simulink model "DecoupledControl"  (R2022a)
settings: Solver=VariableStepAuto  StartTime=0.0  StopTime=30  MaxStep=0.0001  RelTol=1e-3
undefined symbols (not defined in the file): K1, K2, N1, N2, q01, q02, tau0
settings Model: Creator=y.briere  LastModifiedBy=fades
settings DebuggingCC: UnconnectedInputMsg=warning  UnconnectedOutputMsg=warning  UnconnectedLineMsg=warning
settings RTWCC: DLArmComputeVersion=19.05

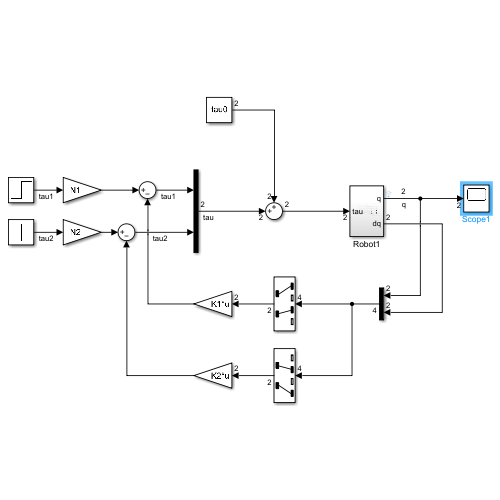
[thumbnail: Simulink's stored preview of the top-level diagram]
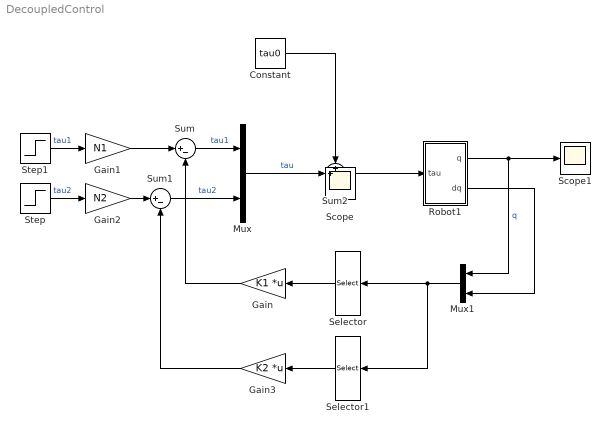
== system DecoupledControl ==
  Constant : Constant  Value=tau0
  Gain : Gain  Gain=K1  Multiplication=Matrix(K*u)
  Gain1 : Gain  Gain=N1
  Gain2 : Gain  Gain=N2
  Gain3 : Gain  Gain=K2  Multiplication=Matrix(K*u)
  Mux : Mux  Inputs=2
  Mux1 : Mux  Inputs=2
  Robot1 : Subsystem
  Scope1 : Scope
  Selector : Selector  InputPortWidth=4  IndexOptions=Index vector (dialog)  Indices=[1 3]  OutputSizes=1
  Selector1 : Selector  InputPortWidth=4  IndexOptions=Index vector (dialog)  Indices=[2 4]  OutputSizes=1
  Step : Step  Time=10  Before=q02  After=q02 + pi/2  SampleTime=0
  Step1 : Step  Before=q01  After=q01  SampleTime=0
  Sum : Sum  Inputs=|+-
  Sum1 : Sum  Inputs=|+-
  Sum2 : Sum  Inputs=++|
  Scope : Scope
  wires:
  Sum1/1 -> Mux/2  "tau2"
  Sum/1 -> Mux/1  "tau1"
  Robot1/1(q) -> Mux1/1, Scope1/1  "q"
  Selector/1 -> Gain/1
  Step1/1 -> Gain1/1  "tau1"
  Step/1 -> Gain2/1  "tau2"
  Gain2/1 -> Sum1/1
  Selector1/1 -> Gain3/1
  Gain/1 -> Sum/2
  Gain3/1 -> Sum1/2
  Mux1/1 -> Selector1/1, Selector/1
  Robot1/2(dq) -> Mux1/2
  Gain1/1 -> Sum/1
  Constant/1 -> Sum2/1
  Sum2/1 -> Robot1/1(tau)
  Mux/1 -> Sum2/2  "tau"

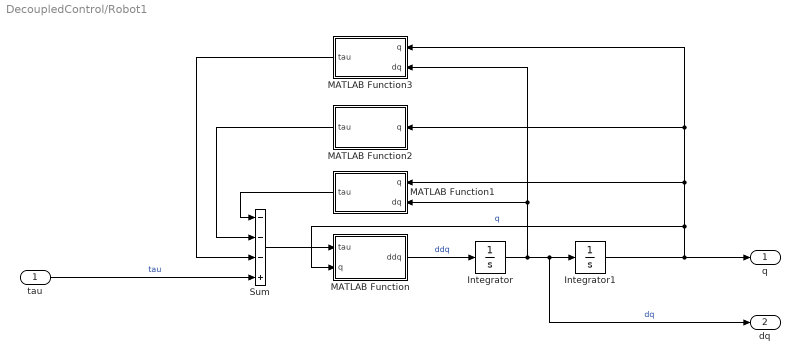
== system DecoupledControl/Robot1 ==
  tau : Inport
  Integrator : Integrator  InitialCondition=[0:0]
  Integrator1 : Integrator  InitialCondition=[q01;q02]
  MATLAB Function : MATLAB Function  TreatAsAtomicUnit=on
  MATLAB Function1 : MATLAB Function  TreatAsAtomicUnit=on
  MATLAB Function2 : MATLAB Function  TreatAsAtomicUnit=on
  MATLAB Function3 : MATLAB Function  TreatAsAtomicUnit=on
  Sum : Sum  Inputs=---+
  q : Outport
  dq : Outport  Port=2
  wires:
  Integrator/1 -> MATLAB Function3/2(dq), MATLAB Function1/2(dq), dq/1, Integrator1/1  "dq"
  Integrator1/1 -> MATLAB Function3/1(q), MATLAB Function2/1(q), MATLAB Function1/1(q), MATLAB Function/2(q), q/1  "q"
  MATLAB Function3/1(tau) -> Sum/3
  MATLAB Function/1(ddq) -> Integrator/1  "ddq"
  Sum/1 -> MATLAB Function/1(tau)
  MATLAB Function1/1(tau) -> Sum/1
  MATLAB Function2/1(tau) -> Sum/2
  tau/1 -> Sum/4  "tau"

== matlab function DecoupledControl/Robot1/MATLAB Function ==
  data: tau input; q input; ddq output
function ddq  = invM(tau,q)
% Mass matrix
R.m1 = 1; % Arm 1 mass
R.m2 = 1; % Arm 2 mass
R.L1 = 1; % Arm 1 length
R.L2 = 1; % Arm 2 length
M = [(R.m1*R.L1^2)/4+R.m2*(R.L1^2+R.L2^2/4+R.L1*R.L2*cos(q(2))) ,  R.m2*R.L2*(R.L2+ 2*R.L1*cos(q(2)))/4
    R.m2*R.L2*(R.L2+ 2*R.L1*cos(q(2)))/4                       ,  R.m2*R.L2^2/4];

ddq = M\tau;

== matlab function DecoupledControl/Robot1/MATLAB Function1 ==
  data: q input; dq input; tau output
function tau  = coriolis(q,dq)
% Convective Matrix
%Robot parameters
R.m1 = 1; % Arm 1 mass
R.m2 = 1; % Arm 2 mass
R.L1 = 1; % Arm 1 length
R.L2 = 1; % Arm 2 length
Cm = [-R.m2*R.L1*R.L2*sin(q(2))*dq(2) -R.m2*R.L1*R.L2*sin(q(2))/2*dq(2);...
    R.m2*R.L1*R.L2*dq(1)*sin(q(2))/2 0];
tau = Cm*dq;

== matlab function DecoupledControl/Robot1/MATLAB Function2 ==
  data: q input; tau output
function tau  = gravity(q)
%Robot parameters
R.m1 = 1; % Arm 1 mass
R.m2 = 1; % Arm 2 mass
R.L1 = 1; % Arm 1 length
R.L2 = 1; % Arm 2 length
R.g = 0*9.81; % Gravity

tau = [R.m1*R.g*R.L1*cos(q(1))/2+R.m2*R.g*(R.L2*cos(q(1)+q(2))/2+R.L1*cos(q(1)));...
    R.m2*R.g*R.L2*cos(q(1)+q(2))/2];

== matlab function DecoupledControl/Robot1/MATLAB Function3 ==
  data: q input; dq input; tau output
function tau  = friction(q,dq)
%Robot parameters
R.f1 = 1; % Friction 1
R.f2 = 1; % Friction 2

tau = [R.f1
    R.f2].*dq;
